simulink model "CNL_TP1_SysLinSaturation_SimuLink_editd"  (R2020a)
settings: Solver=VariableStepAuto  StartTime=0.0  StopTime=10.0  RelTol=1e-10
settings Model: Creator=damie  LastModifiedBy=damie

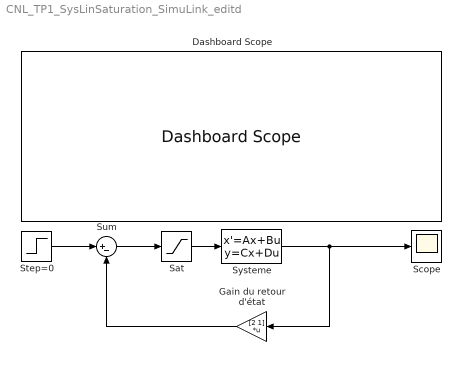
== system CNL_TP1_SysLinSaturation_SimuLink_editd ==
  Dashboard Scope : DashboardScope
  Gain du retour d'état : Gain  Gain=[2 1]  Multiplication=Matrix(K*u)
  Sat : Saturate  UpperLimit=1  LowerLimit=-1
  Scope : Scope
  Step=0 : Step  After=0  SampleTime=0
  Sum : Sum  Inputs=|+-
  Systeme : StateSpace  A=[0 1; 1 0]  B=[0; 1]  C=eye(2)  D=[0;0]  InitialCondition=[0;2]
  wires:
  Systeme/1 -> Gain du retour d'état/1, Scope/1
  Sat/1 -> Systeme/1
  Step=0/1 -> Sum/1
  Sum/1 -> Sat/1
  Gain du retour d'état/1 -> Sum/2
